simulink model "AariaJoystickR2017a"  (R2017a)
settings: Solver=VariableStepAuto  StartTime=0.0  StopTime=inf  FixedStep=0.1  RelTol=1e-3  EnableMultiTasking=on
model workspace (MATLAB code in the model file):
  | my_a =1;
undefined symbols (not defined in the file or in its folder): AARIAENV, AARIAMAN, AARIASEN, Camera, sensor, Source_TS, X, Y, Z
libraries: sm_lib x723, nesl_utility x640, dspmathops x314, simulink x168, vrlib x2, powerlib_meascontrol x1, aerolibanimutils x1, aerolibutil x1
(part 2 of 26)

== system AariaJoystickR2017a/Tool ==
  Cam_vis : sm_lib/Body Elements/Solid  InertiaType=CalculateFromGeometry  Mass=0  MassUnits=kg  CenterOfMass=[0 0 0]  CenterOfMassUnits=m  MomentsOfInertia=[1 1 1]  MomentsOfInertiaUnits=kg*m^2  ProductsOfInertia=[1 1 1]  ProductsOfInertiaUnits=kg*m^2  DensityBased=off  Density=1000  DensityUnits=kg/m^3  DoExposeReferenceFrame=on  SerializedFrames=<Frames/>  GraphicType=FromGeometry  MarkerShape=Sphere  MarkerSize=10  GraphicVisPropType=SimpleVisualProperties  GraphicDiffuseColor=[0.5 0.5 0.5]  GraphicSpecularColor=[0.5 0.5 0.5 1.0]  GraphicAmbientColor=[0.15 0.15 0.15 1.0]  GraphicEmissiveColor=[0.0 0.0 0.0 1.0]  GraphicShininess=75  GraphicOpacity=1.0  GeometryShape=Sphere  RectangleSize=[1 1]  RectangleSizeUnits=m  BrickDimensions=[0.01 0.01 0.2]  BrickDimensionUnits=m  CylinderRadius=1  CylinderRadiusUnits=m  CylinderLength=1  CylinderLengthUnits=m  SphereRadius=0.02  SphereRadiusUnits=m  EllipsoidRadii=[1 1 1]  EllipsoidRadiiUnits=m  ExtrusionCrossSection=[1 1; -1 1; -1 -1; 1 -1]  ExtrusionCrossSectionUnits=m  ExtrusionLength=1  ExtrusionLengthUnits=m  PolygonNumSides=3  PolygonOuterRadius=1  PolygonOuterRadiusUnits=m  ExtGeomFileType=STEP  ExtGeomFileUnits=m  RevolutionCrossSection=[1 1; 1 -1; 2 -1; 2 1]  RevolutionCrossSectionUnits=m  RevolutionExtent=Full  RevolutionAngle=180  RevolutionAngleUnits=deg
  Camera : sm_lib/Frames and Transforms/Reference Frame
  Coord_ToolTip : sm_lib/Body Elements/Graphic  GraphicType=Marker  MarkerShape=Frame  MarkerSize=AARIAMAN.vis.coord_size  GraphicVisPropType=SimpleVisualProperties  GraphicDiffuseColor=[1.0 1.0 0.0]  GraphicSpecularColor=[0.5 0.5 0.5 1.0]  GraphicAmbientColor=[0.15 0.15 0.15 1.0]  GraphicEmissiveColor=[0.0 0.0 0.0 1.0]  GraphicShininess=75  GraphicOpacity=1.0
      settings: SourceProductName=Simscape Multibody
  IMU Tool : Subsystem  mask{nL=Link_number}
      mask prompts: nL "Link Number (nL)"
      mask DialogControl DescTextVar Prompt: A Set of IMUs for one body
  Mux : Mux  Inputs=2
  Rigid Transform : sm_lib/Frames and Transforms/Rigid Transform  TranslationMethod=None  TranslationStandardOffset=0  TranslationLengthUnit=m  TranslationStandardAxis=+Z  TranslationCartesianOffset=[0 0 0]  TranslationROffset=0  TranslationROffsetUnits=m  TranslationZOffset=0  TranslationZOffsetUnits=m  TranslationThetaOffset=0  TranslationThetaOffsetUnits=deg  RotationMethod=AlignedAxes  RotationAngleUnits=deg  RotationStandardAxis=+Z  RotationAngle=0.0  RotationArbitraryAxis=[0 0 1]  FollAlignAxisA=+X  BaseAlignAxisA=+Z  FollAlignAxisB=+Z  BaseAlignAxisB=+Y  RotationSequenceAxes=FollowerAxes  RotationSequence=XYX  RotationSequenceAngles=[0 0 0]  RotationSequenceAnglesUnits=deg  RotationMatrix=[1 0 0; 0 1 0; 0 0 1]
  Rigid Transform1 : sm_lib/Frames and Transforms/Rigid Transform  TranslationMethod=StandardAxis  TranslationStandardOffset=AARIAMAN.DH(Link_number).a/2  TranslationLengthUnit=m  TranslationStandardAxis=+Z  TranslationCartesianOffset=0.1  TranslationROffset=0  TranslationROffsetUnits=m  TranslationZOffset=0  TranslationZOffsetUnits=m  TranslationThetaOffset=0  TranslationThetaOffsetUnits=deg  RotationMethod=None  RotationAngleUnits=deg  RotationStandardAxis=+Z  RotationAngle=0.0  RotationArbitraryAxis=[0 0 1]  FollAlignAxisA=+X  BaseAlignAxisA=+Y  FollAlignAxisB=+Y  BaseAlignAxisB=+Z  RotationSequenceAxes=FollowerAxes  RotationSequence=XYX  RotationSequenceAngles=[0 0 0]  RotationSequenceAnglesUnits=deg  RotationMatrix=[1 0 0; 0 1 0; 0 0 1]
  Rigid Transform2 : sm_lib/Frames and Transforms/Rigid Transform  TranslationMethod=StandardAxis  TranslationStandardOffset=AARIAMAN.DH(Link_number).a/2  TranslationLengthUnit=m  TranslationStandardAxis=+Z  TranslationCartesianOffset=0.1  TranslationROffset=0  TranslationROffsetUnits=m  TranslationZOffset=0  TranslationZOffsetUnits=m  TranslationThetaOffset=0  TranslationThetaOffsetUnits=deg  RotationMethod=None  RotationAngleUnits=deg  RotationStandardAxis=+Z  RotationAngle=0.0  RotationArbitraryAxis=[0 0 1]  FollAlignAxisA=+X  BaseAlignAxisA=+Y  FollAlignAxisB=+Y  BaseAlignAxisB=+Z  RotationSequenceAxes=FollowerAxes  RotationSequence=XYX  RotationSequenceAngles=[0 0 0]  RotationSequenceAnglesUnits=deg  RotationMatrix=[1 0 0; 0 1 0; 0 0 1]
  Rigid Transform3 : sm_lib/Frames and Transforms/Rigid Transform  TranslationMethod=StandardAxis  TranslationStandardOffset=AARIAMAN.DH(Link_number).d-0.01  TranslationLengthUnit=m  TranslationStandardAxis=-X  TranslationCartesianOffset=0.1  TranslationROffset=0  TranslationROffsetUnits=m  TranslationZOffset=0  TranslationZOffsetUnits=m  TranslationThetaOffset=0  TranslationThetaOffsetUnits=deg  RotationMethod=None  RotationAngleUnits=deg  RotationStandardAxis=+Z  RotationAngle=0.0  RotationArbitraryAxis=[0 0 1]  FollAlignAxisA=+X  BaseAlignAxisA=+Y  FollAlignAxisB=+Y  BaseAlignAxisB=+Z  RotationSequenceAxes=FollowerAxes  RotationSequence=XYX  RotationSequenceAngles=[0 0 0]  RotationSequenceAnglesUnits=deg  RotationMatrix=[1 0 0; 0 1 0; 0 0 1]
  Rigid Transform4 : sm_lib/Frames and Transforms/Rigid Transform  TranslationMethod=None  TranslationStandardOffset=0  TranslationLengthUnit=m  TranslationStandardAxis=+Z  TranslationCartesianOffset=[0 0 0]  TranslationROffset=0  TranslationROffsetUnits=m  TranslationZOffset=0  TranslationZOffsetUnits=m  TranslationThetaOffset=0  TranslationThetaOffsetUnits=deg  RotationMethod=AlignedAxes  RotationAngleUnits=deg  RotationStandardAxis=+Z  RotationAngle=0.0  RotationArbitraryAxis=[0 0 1]  FollAlignAxisA=+X  BaseAlignAxisA=+Z  FollAlignAxisB=+Z  BaseAlignAxisB=+Y  RotationSequenceAxes=FollowerAxes  RotationSequence=XYX  RotationSequenceAngles=[0 0 0]  RotationSequenceAnglesUnits=deg  RotationMatrix=[1 0 0; 0 1 0; 0 0 1]
  Rigid Transform5 : sm_lib/Frames and Transforms/Rigid Transform  TranslationMethod=None  TranslationStandardOffset=0.1  TranslationLengthUnit=m  TranslationStandardAxis=+Y  TranslationCartesianOffset=[0 0 0]  TranslationROffset=0  TranslationROffsetUnits=m  TranslationZOffset=0  TranslationZOffsetUnits=m  TranslationThetaOffset=0  TranslationThetaOffsetUnits=deg  RotationMethod=RotationMatrix  RotationAngleUnits=rad  RotationStandardAxis=+X  RotationAngle=Camera.Rotation  RotationArbitraryAxis=[0 0 1]  FollAlignAxisA=+X  BaseAlignAxisA=+Y  FollAlignAxisB=+Y  BaseAlignAxisB=+Z  RotationSequenceAxes=FollowerAxes  RotationSequence=XYX  RotationSequenceAngles=[0 0 0]  RotationSequenceAnglesUnits=deg  RotationMatrix=Camera.Rotation
  Rigid Transform7 : sm_lib/Frames and Transforms/Rigid Transform  TranslationMethod=Cartesian  TranslationStandardOffset=0.1  TranslationLengthUnit=m  TranslationStandardAxis=+Y  TranslationCartesianOffset=Camera.Offset  TranslationROffset=0  TranslationROffsetUnits=m  TranslationZOffset=0  TranslationZOffsetUnits=m  TranslationThetaOffset=0  TranslationThetaOffsetUnits=deg  RotationMethod=None  RotationAngleUnits=rad  RotationStandardAxis=+X  RotationAngle=Camera.Rotation  RotationArbitraryAxis=[0 0 1]  FollAlignAxisA=+X  BaseAlignAxisA=+Y  FollAlignAxisB=+Y  BaseAlignAxisB=+Z  RotationSequenceAxes=FollowerAxes  RotationSequence=XYX  RotationSequenceAngles=[0 0 0]  RotationSequenceAnglesUnits=deg  RotationMatrix=[1 0 0; 0 1 0; 0 0 1]
  Rigid Transform8 : sm_lib/Frames and Transforms/Rigid Transform  TranslationMethod=StandardAxis  TranslationStandardOffset=Camera.ObjectRadius  TranslationLengthUnit=m  TranslationStandardAxis=+Z  TranslationCartesianOffset=Camera.Offset  TranslationROffset=0  TranslationROffsetUnits=m  TranslationZOffset=0  TranslationZOffsetUnits=m  TranslationThetaOffset=0  TranslationThetaOffsetUnits=deg  RotationMethod=None  RotationAngleUnits=deg  RotationStandardAxis=+X  RotationAngle=-90  RotationArbitraryAxis=[0 0 1]  FollAlignAxisA=+X  BaseAlignAxisA=+Y  FollAlignAxisB=+Y  BaseAlignAxisB=+Z  RotationSequenceAxes=FollowerAxes  RotationSequence=XYX  RotationSequenceAngles=[0 0 0]  RotationSequenceAnglesUnits=deg  RotationMatrix=0
  Rigid Transform9 : sm_lib/Frames and Transforms/Rigid Transform  TranslationMethod=StandardAxis  TranslationStandardOffset=AARIAMAN.DH(Link_number).d-0.01  TranslationLengthUnit=m  TranslationStandardAxis=+X  TranslationCartesianOffset=0.1  TranslationROffset=0  TranslationROffsetUnits=m  TranslationZOffset=0  TranslationZOffsetUnits=m  TranslationThetaOffset=0  TranslationThetaOffsetUnits=deg  RotationMethod=None  RotationAngleUnits=deg  RotationStandardAxis=+Z  RotationAngle=0.0  RotationArbitraryAxis=[0 0 1]  FollAlignAxisA=+X  BaseAlignAxisA=+Y  FollAlignAxisB=+Y  BaseAlignAxisB=+Z  RotationSequenceAxes=FollowerAxes  RotationSequence=XYX  RotationSequenceAngles=[0 0 0]  RotationSequenceAnglesUnits=deg  RotationMatrix=[1 0 0; 0 1 0; 0 0 1]
  Terminator : Terminator
  Terminator1 : Terminator
  ToDH : sm_lib/Frames and Transforms/Rigid Transform  TranslationMethod=None  TranslationStandardOffset=0  TranslationLengthUnit=m  TranslationStandardAxis=+Z  TranslationCartesianOffset=[0 0 0]  TranslationROffset=0  TranslationROffsetUnits=m  TranslationZOffset=0  TranslationZOffsetUnits=m  TranslationThetaOffset=0  TranslationThetaOffsetUnits=deg  RotationMethod=RotationMatrix  RotationAngleUnits=deg  RotationStandardAxis=+Z  RotationAngle=0.0  RotationArbitraryAxis=[0 0 1]  FollAlignAxisA=+X  BaseAlignAxisA=+Y  FollAlignAxisB=+Y  BaseAlignAxisB=+Z  RotationSequenceAxes=FollowerAxes  RotationSequence=XYX  RotationSequenceAngles=[0 0 0]  RotationSequenceAnglesUnits=deg  RotationMatrix=AARIAMAN.L(Link_number).toDH
  Tool : sm_lib/Body Elements/Solid  InertiaType=CalculateFromGeometry  Mass=abs(AARIAMAN.L(Link_number).massLink)  MassUnits=kg  CenterOfMass=[0 0 0]  CenterOfMassUnits=m  MomentsOfInertia=[1 1 1]  MomentsOfInertiaUnits=kg*m^2  ProductsOfInertia=[0 0 0]  ProductsOfInertiaUnits=kg*m^2  DensityBased=off  Density=1000  DensityUnits=kg/(m^3)  DoExposeReferenceFrame=on  SerializedFrames=<Frames/>  GraphicType=FromGeometry  MarkerShape=Sphere  MarkerSize=10  GraphicVisPropType=SimpleVisualProperties  GraphicDiffuseColor=[0.6 0.0 0.0]  GraphicSpecularColor=[0.5 0.5 0.5 1.0]  GraphicAmbientColor=[0.15 0.15 0.15 1.0]  GraphicEmissiveColor=[0.0 0.0 0.0 1.0]  GraphicShininess=75  GraphicOpacity=AARIAMAN.L(Link_number).linkOpacity  GeometryShape=Cylinder  RectangleSize=[1 1]  RectangleSizeUnits=m  BrickDimensions=[1 1 1]  BrickDimensionUnits=m  CylinderRadius=abs(AARIAMAN.DH(Link_number).d)+0.001  CylinderRadiusUnits=m  CylinderLength=AARIAMAN.DH(Link_number).a+0.001  CylinderLengthUnits=m  SphereRadius=1  SphereRadiusUnits=m  EllipsoidRadii=[1 1 1]  EllipsoidRadiiUnits=m  ExtrusionCrossSection=[1 1; -1 1; -1 -1; 1 -1]  ExtrusionCrossSectionUnits=m  ExtrusionLength=1  ExtrusionLengthUnits=m  PolygonNumSides=3  PolygonOuterRadius=1  PolygonOuterRadiusUnits=m  ExtGeomFileType=STL  ExtGeomFileUnits=m  RevolutionCrossSection=[1 1; 1 -1; 2 -1; 2 1]  RevolutionCrossSectionUnits=m  RevolutionExtent=Full  RevolutionAngle=180  RevolutionAngleUnits=deg
  Tool1 : sm_lib/Body Elements/Solid  InertiaType=CalculateFromGeometry  Mass=AARIAMAN.vis.joint_mass/10  MassUnits=kg  CenterOfMass=[0 0 0]  CenterOfMassUnits=m  MomentsOfInertia=[1 1 1]  MomentsOfInertiaUnits=kg*m^2  ProductsOfInertia=[0 0 0]  ProductsOfInertiaUnits=kg*m^2  DensityBased=off  Density=1000  DensityUnits=kg/(m^3)  DoExposeReferenceFrame=on  SerializedFrames=<Frames/>  GraphicType=FromGeometry  MarkerShape=Sphere  MarkerSize=10  GraphicVisPropType=SimpleVisualProperties  GraphicDiffuseColor=[0.6 0.0 0.0]  GraphicSpecularColor=[0.5 0.5 0.5 1.0]  GraphicAmbientColor=[0.15 0.15 0.15 1.0]  GraphicEmissiveColor=[0.0 0.0 0.0 1.0]  GraphicShininess=75  GraphicOpacity=1.0  GeometryShape=Brick  RectangleSize=[1 1]  RectangleSizeUnits=m  BrickDimensions=[0.01 0.1 0.1]  BrickDimensionUnits=m  CylinderRadius=1  CylinderRadiusUnits=m  CylinderLength=1  CylinderLengthUnits=m  SphereRadius=1  SphereRadiusUnits=m  EllipsoidRadii=[1 1 1]  EllipsoidRadiiUnits=m  ExtrusionCrossSection=[1 1; -1 1; -1 -1; 1 -1]  ExtrusionCrossSectionUnits=m  ExtrusionLength=1  ExtrusionLengthUnits=m  PolygonNumSides=4  PolygonOuterRadius=1  PolygonOuterRadiusUnits=m  ExtGeomFileType=STL  ExtGeomFileUnits=m  RevolutionCrossSection=[1 1; 1 -1; 2 -1; 2 1]  RevolutionCrossSectionUnits=m  RevolutionExtent=Full  RevolutionAngle=180  RevolutionAngleUnits=deg
  Tool2 : sm_lib/Body Elements/Solid  InertiaType=CalculateFromGeometry  Mass=AARIAMAN.vis.joint_mass/10  MassUnits=kg  CenterOfMass=[0 0 0]  CenterOfMassUnits=m  MomentsOfInertia=[1 1 1]  MomentsOfInertiaUnits=kg*m^2  ProductsOfInertia=[0 0 0]  ProductsOfInertiaUnits=kg*m^2  DensityBased=off  Density=1000  DensityUnits=kg/(m^3)  DoExposeReferenceFrame=on  SerializedFrames=<Frames/>  GraphicType=FromGeometry  MarkerShape=Sphere  MarkerSize=10  GraphicVisPropType=SimpleVisualProperties  GraphicDiffuseColor=[0.6 0.0 0.0]  GraphicSpecularColor=[0.5 0.5 0.5 1.0]  GraphicAmbientColor=[0.15 0.15 0.15 1.0]  GraphicEmissiveColor=[0.0 0.0 0.0 1.0]  GraphicShininess=75  GraphicOpacity=1.0  GeometryShape=Brick  RectangleSize=[1 1]  RectangleSizeUnits=m  BrickDimensions=[0.01 0.1 0.1]  BrickDimensionUnits=m  CylinderRadius=1  CylinderRadiusUnits=m  CylinderLength=1  CylinderLengthUnits=m  SphereRadius=1  SphereRadiusUnits=m  EllipsoidRadii=[1 1 1]  EllipsoidRadiiUnits=m  ExtrusionCrossSection=[1 1; -1 1; -1 -1; 1 -1]  ExtrusionCrossSectionUnits=m  ExtrusionLength=1  ExtrusionLengthUnits=m  PolygonNumSides=4  PolygonOuterRadius=1  PolygonOuterRadiusUnits=m  ExtGeomFileType=STL  ExtGeomFileUnits=m  RevolutionCrossSection=[1 1; 1 -1; 2 -1; 2 1]  RevolutionCrossSectionUnits=m  RevolutionExtent=Full  RevolutionAngle=180  RevolutionAngleUnits=deg
  force_torque_sensor : Subsystem
  Base : PMIOPort  Port=1  Side=Left
  Reference : PMIOPort  Port=2  Side=Left
  Cam : PMIOPort  Port=3  Side=Right
  ToolTip : PMIOPort  Port=4  Side=Right
  Out1 : Outport
  Tool_torque : Outport  Port=2
  wires:
  IMU Tool/1(Out1) -> Mux/1
  IMU Tool/2(Out2) -> Mux/2
  Mux/1 -> Out1/1
  IMU Tool/3(Out3) -> Terminator/1
  IMU Tool/4(Out4) -> Terminator1/1
  force_torque_sensor/1(XYZ_force_torque) -> Tool_torque/1
  connections:
  Rigid Transform1/RConn1 -- Rigid Transform2/LConn1 -- Tool/RConn1
  IMU Tool/LConn2 -- Reference/RConn1
  ToDH/RConn1 -- Rigid Transform1/LConn1
  force_torque_sensor/LConn1 -- Base/RConn1
  force_torque_sensor/RConn1 -- ToDH/LConn1
  Rigid Transform9/LConn1 -- Rigid Transform3/LConn1 -- Rigid Transform7/LConn1 -- Rigid Transform8/LConn1 -- IMU Tool/LConn1 -- Rigid Transform2/RConn1
  Rigid Transform3/RConn1 -- Tool2/RConn1
  Tool1/RConn1 -- Rigid Transform9/RConn1
  Coord_ToolTip/RConn1 -- ToolTip/RConn1 -- Rigid Transform/RConn1
  Cam/RConn1 -- Rigid Transform5/RConn1 -- Cam_vis/RConn1 -- Camera/RConn1
  Rigid Transform/LConn1 -- Rigid Transform8/RConn1
  Rigid Transform4/RConn1 -- Rigid Transform5/LConn1
  Rigid Transform4/LConn1 -- Rigid Transform7/RConn1

== system AariaJoystickR2017a/Tool Sensors ==
  Camera sensor : Subsystem
  Object tracker : Subsystem
  Terminator{,1..5,8} (7 alike) : Terminator
  Tool sensor1 : Subsystem
  Tool sensor2 : Subsystem
  Camera : PMIOPort  Port=1  Side=Left
  ToolTip : PMIOPort  Port=2  Side=Left
  World : PMIOPort  Port=3  Side=Left
  Object : PMIOPort  Port=4  Side=Left
  cam2tip2sph : Outport
  SphericalRad : Outport  Port=2
  ObjPose : Outport  Port=3
  tipxyz1 : Outport  Port=4
  rot axis : Outport  Port=5
  Rmat : Outport  Port=6
  Omega : Outport  Port=7
  wires:
  Camera sensor/1(Out3) -> Object tracker/1(CamRotation)
  Tool sensor2/3(Out2) -> cam2tip2sph/1
  Camera sensor/2(Out1) -> Terminator/1
  Camera sensor/3(Out2) -> Terminator1/1
  Tool sensor2/1(Out3) -> Terminator2/1
  Tool sensor2/2(Out1) -> Terminator3/1
  Object tracker/1(Spherical Rad) -> SphericalRad/1
  Object tracker/2(Obj_pose) -> ObjPose/1
  Object tracker/3(Obj_pose_world) -> Terminator4/1
  Object tracker/4(xyz_true) -> Terminator5/1
  Tool sensor1/2(Out1) -> tipxyz1/1
  Tool sensor1/1(Out3) -> Rmat/1
  Tool sensor1/3(Out2) -> Terminator8/1
  Tool sensor1/4(rot axis) -> rot axis/1
  Tool sensor1/5(Omega) -> Omega/1
  connections:
  World/RConn1 -- Tool sensor1/LConn2 -- Camera sensor/LConn2
  Camera/RConn1 -- Tool sensor2/LConn2 -- Object tracker/LConn1 -- Camera sensor/LConn1
  Object/RConn1 -- Object tracker/RConn1
  Tool sensor2/LConn1 -- Tool sensor1/LConn1 -- ToolTip/RConn1

== system AariaJoystickR2017a/Base/BaseVSS ==
  BaseEmpty : Subsystem  VariantControl=VSS_MODE8 == 0
  BaseMotion : Subsystem  VariantControl=VSS_MODE8 == 1
  BaseTorque : Subsystem  VariantControl=VSS_MODE8 == 2
  Start : PMIOPort  Port=1  Side=Left
  End : PMIOPort  Port=2  Side=Right
  IMU : Outport

== system AariaJoystickR2017a/Joint1/JointVSS ==
  Control : Inport
  Empty : Subsystem  VariantControl=VSS_MODE1 == 0
  PrismaticMotion : Subsystem  VariantControl=VSS_MODE1 == 2
  PrismaticTorque : Subsystem  VariantControl=VSS_MODE1 == 4
  RevoluteMotion : Subsystem  VariantControl=VSS_MODE1 == 1
  RevoluteTorque : Subsystem  VariantControl=VSS_MODE1 == 3
  Start : PMIOPort  Port=1  Side=Left
  End : PMIOPort  Port=2  Side=Right
  Reference coord : PMIOPort  Port=3  Side=Left
  IMU : Outport
  Joint : Outport  Port=2

== system AariaJoystickR2017a/Joint2/JointVSS ==
  Control : Inport
  Empty : Subsystem  VariantControl=VSS_MODE2 == 0
  PrismaticMotion : Subsystem  VariantControl=VSS_MODE2 == 2
  PrismaticTorque : Subsystem  VariantControl=VSS_MODE2 == 4
  RevoluteMotion : Subsystem  VariantControl=VSS_MODE2 == 1
  RevoluteTorque : Subsystem  VariantControl=VSS_MODE2 == 3
  Start : PMIOPort  Port=1  Side=Left
  End : PMIOPort  Port=2  Side=Right
  Reference coord : PMIOPort  Port=3  Side=Left
  IMU : Outport
  Joint : Outport  Port=2

== system AariaJoystickR2017a/Joint3/JointVSS ==
  Control : Inport
  Empty : Subsystem  VariantControl=VSS_MODE3 == 0
  PrismaticMotion : Subsystem  VariantControl=VSS_MODE3 == 2
  PrismaticTorque : Subsystem  VariantControl=VSS_MODE3 == 4
  RevoluteMotion : Subsystem  VariantControl=VSS_MODE3 == 1
  RevoluteTorque : Subsystem  VariantControl=VSS_MODE3 == 3
  Start : PMIOPort  Port=1  Side=Left
  End : PMIOPort  Port=2  Side=Right
  Reference coord : PMIOPort  Port=3  Side=Left
  IMU : Outport
  Joint : Outport  Port=2

== system AariaJoystickR2017a/Joint4/JointVSS ==
  Control : Inport
  Empty : Subsystem  VariantControl=VSS_MODE4 == 0
  PrismaticMotion : Subsystem  VariantControl=VSS_MODE4 == 2
  PrismaticTorque : Subsystem  VariantControl=VSS_MODE4 == 4
  RevoluteMotion : Subsystem  VariantControl=VSS_MODE4 == 1
  RevoluteTorque : Subsystem  VariantControl=VSS_MODE4 == 3
  Start : PMIOPort  Port=1  Side=Left
  End : PMIOPort  Port=2  Side=Right
  Reference coord : PMIOPort  Port=3  Side=Left
  IMU : Outport
  Joint : Outport  Port=2

== system AariaJoystickR2017a/Joint5/JointVSS ==
  Control : Inport
  Empty : Subsystem  VariantControl=VSS_MODE5 == 0
  PrismaticMotion : Subsystem  VariantControl=VSS_MODE5 == 2
  PrismaticTorque : Subsystem  VariantControl=VSS_MODE5 == 4
  RevoluteMotion : Subsystem  VariantControl=VSS_MODE5 == 1
  RevoluteTorque : Subsystem  VariantControl=VSS_MODE5 == 3
  Start : PMIOPort  Port=1  Side=Left
  End : PMIOPort  Port=2  Side=Right
  Reference coord : PMIOPort  Port=3  Side=Left
  IMU : Outport
  Joint : Outport  Port=2

== system AariaJoystickR2017a/Joint6/JointVSS ==
  Control : Inport
  Empty : Subsystem  VariantControl=VSS_MODE6 == 0
  PrismaticMotion : Subsystem  VariantControl=VSS_MODE6 == 2
  PrismaticTorque : Subsystem  VariantControl=VSS_MODE6 == 4
  RevoluteMotion : Subsystem  VariantControl=VSS_MODE6 == 1
  RevoluteTorque : Subsystem  VariantControl=VSS_MODE6 == 3
  Start : PMIOPort  Port=1  Side=Left
  End : PMIOPort  Port=2  Side=Right
  Reference coord : PMIOPort  Port=3  Side=Left
  IMU : Outport
  Joint : Outport  Port=2

== system AariaJoystickR2017a/JoystickInputs/Variant Subsystem ==
  note: 1) Add Subsystem or Model blocks as valid variant choices.
      | 2) You cannot connect blocks at this level. At simulation, connectivity is automatically
      | determined, based on the active variant and port name matching.
  VSS_Live : Subsystem  VariantControl=VSS_Joystick == 1
  VSS_Replay : Subsystem  VariantControl=VSS_Joystick == 2
  Out1 : Outport
  Out2 : Outport  Port=2
  Out3 : Outport  Port=3
  Out4 : Outport  Port=4
  Out5 : Outport  Port=5
  Out6 : Outport  Port=6
  Out7 : Outport  Port=7

== system AariaJoystickR2017a/JoystickInputs/Variant Subsystem1 ==
  note: 1) Add Subsystem or Model blocks as valid variant choices.
      | 2) You cannot connect blocks at this level. At simulation, connectivity is automatically
      | determined, based on the active variant and port name matching.
  VSS_Live : Subsystem  VariantControl=VSS_Joystick == 1
  VSS_Replay : Subsystem  VariantControl=VSS_Joystick == 2
  Out1 : Outport
  Out2 : Outport  Port=2
  Out3 : Outport  Port=3
  Out4 : Outport  Port=4
  Out5 : Outport  Port=5
  Out6 : Outport  Port=6
  Out7 : Outport  Port=7

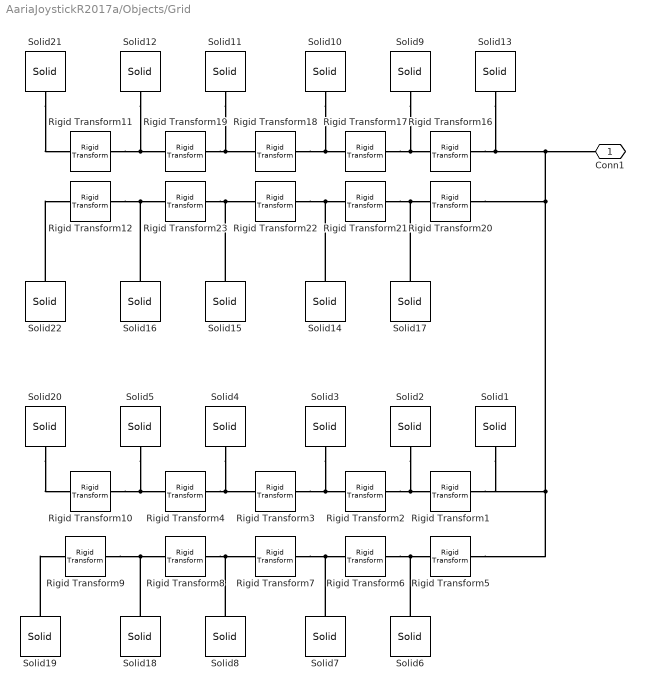
== system AariaJoystickR2017a/Objects/Grid ==
  Rigid Transform{1..4,10} (5 alike) : sm_lib/Frames and Transforms/Rigid Transform  TranslationMethod=StandardAxis  TranslationStandardOffset=2  TranslationLengthUnit=m  TranslationStandardAxis=+Y  TranslationCartesianOffset=[0 0 0]  TranslationROffset=0  TranslationROffsetUnits=m  TranslationZOffset=0  TranslationZOffsetUnits=m  TranslationThetaOffset=0  TranslationThetaOffsetUnits=deg  RotationMethod=None  RotationAngleUnits=deg  RotationStandardAxis=+Z  RotationAngle=0.0  RotationArbitraryAxis=[0 0 1]  FollAlignAxisA=+X  BaseAlignAxisA=+Y  FollAlignAxisB=+Y  BaseAlignAxisB=+Z  RotationSequenceAxes=FollowerAxes  RotationSequence=XYX  RotationSequenceAngles=[0 0 0]  RotationSequenceAnglesUnits=deg  RotationMatrix=[1 0 0; 0 1 0; 0 0 1]
  Rigid Transform{11,16..19} (5 alike) : sm_lib/Frames and Transforms/Rigid Transform  TranslationMethod=StandardAxis  TranslationStandardOffset=2  TranslationLengthUnit=m  TranslationStandardAxis=+X  TranslationCartesianOffset=[0 0 0]  TranslationROffset=0  TranslationROffsetUnits=m  TranslationZOffset=0  TranslationZOffsetUnits=m  TranslationThetaOffset=0  TranslationThetaOffsetUnits=deg  RotationMethod=None  RotationAngleUnits=deg  RotationStandardAxis=+Z  RotationAngle=0.0  RotationArbitraryAxis=[0 0 1]  FollAlignAxisA=+X  BaseAlignAxisA=+Y  FollAlignAxisB=+Y  BaseAlignAxisB=+Z  RotationSequenceAxes=FollowerAxes  RotationSequence=XYX  RotationSequenceAngles=[0 0 0]  RotationSequenceAnglesUnits=deg  RotationMatrix=[1 0 0; 0 1 0; 0 0 1]
  Rigid Transform{12,20..23} (5 alike) : sm_lib/Frames and Transforms/Rigid Transform  TranslationMethod=StandardAxis  TranslationStandardOffset=2  TranslationLengthUnit=m  TranslationStandardAxis=-X  TranslationCartesianOffset=[0 0 0]  TranslationROffset=0  TranslationROffsetUnits=m  TranslationZOffset=0  TranslationZOffsetUnits=m  TranslationThetaOffset=0  TranslationThetaOffsetUnits=deg  RotationMethod=None  RotationAngleUnits=deg  RotationStandardAxis=+Z  RotationAngle=0.0  RotationArbitraryAxis=[0 0 1]  FollAlignAxisA=+X  BaseAlignAxisA=+Y  FollAlignAxisB=+Y  BaseAlignAxisB=+Z  RotationSequenceAxes=FollowerAxes  RotationSequence=XYX  RotationSequenceAngles=[0 0 0]  RotationSequenceAnglesUnits=deg  RotationMatrix=[1 0 0; 0 1 0; 0 0 1]
  Rigid Transform{5..9} (5 alike) : sm_lib/Frames and Transforms/Rigid Transform  TranslationMethod=StandardAxis  TranslationStandardOffset=2  TranslationLengthUnit=m  TranslationStandardAxis=-Y  TranslationCartesianOffset=[0 0 0]  TranslationROffset=0  TranslationROffsetUnits=m  TranslationZOffset=0  TranslationZOffsetUnits=m  TranslationThetaOffset=0  TranslationThetaOffsetUnits=deg  RotationMethod=None  RotationAngleUnits=deg  RotationStandardAxis=+Z  RotationAngle=0.0  RotationArbitraryAxis=[0 0 1]  FollAlignAxisA=+X  BaseAlignAxisA=+Y  FollAlignAxisB=+Y  BaseAlignAxisB=+Z  RotationSequenceAxes=FollowerAxes  RotationSequence=XYX  RotationSequenceAngles=[0 0 0]  RotationSequenceAnglesUnits=deg  RotationMatrix=[1 0 0; 0 1 0; 0 0 1]
  Solid{1..8,18..20} (11 alike) : sm_lib/Body Elements/Solid  InertiaType=CalculateFromGeometry  Mass=1  MassUnits=kg  CenterOfMass=[0 0 0]  CenterOfMassUnits=m  MomentsOfInertia=[1 1 1]  MomentsOfInertiaUnits=kg*m^2  ProductsOfInertia=[1 1 1]  ProductsOfInertiaUnits=kg*m^2  DensityBased=on  Density=1000  DensityUnits=kg/m^3  DoExposeReferenceFrame=on  SerializedFrames=<Frames/>  GraphicType=FromGeometry  MarkerShape=Sphere  MarkerSize=10  GraphicVisPropType=SimpleVisualProperties  GraphicDiffuseColor=[0.4 0.4 0.4]  GraphicSpecularColor=[0.5 0.5 0.5 1.0]  GraphicAmbientColor=[0.15 0.15 0.15 1.0]  GraphicEmissiveColor=[0.0 0.0 0.0 1.0]  GraphicShininess=75  GraphicOpacity=1.0  GeometryShape=Brick  RectangleSize=[1 1]  RectangleSizeUnits=m  BrickDimensions=[20 1 0.12]  BrickDimensionUnits=m  CylinderRadius=1  CylinderRadiusUnits=m  CylinderLength=1  CylinderLengthUnits=m  SphereRadius=1  SphereRadiusUnits=m  EllipsoidRadii=[1 1 1]  EllipsoidRadiiUnits=m  ExtrusionCrossSection=[1 1; -1 1; -1 -1; 1 -1]  ExtrusionCrossSectionUnits=m  ExtrusionLength=1  ExtrusionLengthUnits=m  PolygonNumSides=3  PolygonOuterRadius=1  PolygonOuterRadiusUnits=m  ExtGeomFileType=STEP  ExtGeomFileUnits=m  RevolutionCrossSection=[1 1; 1 -1; 2 -1; 2 1]  RevolutionCrossSectionUnits=m  RevolutionExtent=Full  RevolutionAngle=180  RevolutionAngleUnits=deg
  Solid{9..17,21..22} (11 alike) : sm_lib/Body Elements/Solid  InertiaType=CalculateFromGeometry  Mass=1  MassUnits=kg  CenterOfMass=[0 0 0]  CenterOfMassUnits=m  MomentsOfInertia=[1 1 1]  MomentsOfInertiaUnits=kg*m^2  ProductsOfInertia=[1 1 1]  ProductsOfInertiaUnits=kg*m^2  DensityBased=on  Density=1000  DensityUnits=kg/m^3  DoExposeReferenceFrame=on  SerializedFrames=<Frames/>  GraphicType=FromGeometry  MarkerShape=Sphere  MarkerSize=10  GraphicVisPropType=SimpleVisualProperties  GraphicDiffuseColor=[0.2 0.2 0.2]  GraphicSpecularColor=[0.5 0.5 0.5 1.0]  GraphicAmbientColor=[0.15 0.15 0.15 1.0]  GraphicEmissiveColor=[0.0 0.0 0.0 1.0]  GraphicShininess=75  GraphicOpacity=1.0  GeometryShape=Brick  RectangleSize=[1 1]  RectangleSizeUnits=m  BrickDimensions=[1 20 0.11]  BrickDimensionUnits=m  CylinderRadius=1  CylinderRadiusUnits=m  CylinderLength=1  CylinderLengthUnits=m  SphereRadius=1  SphereRadiusUnits=m  EllipsoidRadii=[1 1 1]  EllipsoidRadiiUnits=m  ExtrusionCrossSection=[1 1; -1 1; -1 -1; 1 -1]  ExtrusionCrossSectionUnits=m  ExtrusionLength=1  ExtrusionLengthUnits=m  PolygonNumSides=3  PolygonOuterRadius=1  PolygonOuterRadiusUnits=m  ExtGeomFileType=STEP  ExtGeomFileUnits=m  RevolutionCrossSection=[1 1; 1 -1; 2 -1; 2 1]  RevolutionCrossSectionUnits=m  RevolutionExtent=Full  RevolutionAngle=180  RevolutionAngleUnits=deg
  Conn1 : PMIOPort  Port=1  Side=Right
  connections:
  Solid12/RConn1 -- Rigid Transform19/RConn1 -- Rigid Transform11/LConn1
  Rigid Transform19/LConn1 -- Solid11/RConn1 -- Rigid Transform18/RConn1
  Rigid Transform16/LConn1 -- Solid13/RConn1 -- Rigid Transform20/LConn1 -- Rigid Transform1/LConn1 -- Solid1/RConn1 -- Rigid Transform5/LConn1 -- Conn1/RConn1
  Rigid Transform21/LConn1 -- Solid17/RConn1 -- Rigid Transform20/RConn1
  Rigid Transform18/LConn1 -- Solid10/RConn1 -- Rigid Transform17/RConn1
  Rigid Transform23/LConn1 -- Rigid Transform22/RConn1 -- Solid15/RConn1
  Rigid Transform22/LConn1 -- Rigid Transform21/RConn1 -- Solid14/RConn1
  Rigid Transform17/LConn1 -- Solid9/RConn1 -- Rigid Transform16/RConn1
  Solid16/RConn1 -- Rigid Transform23/RConn1 -- Rigid Transform12/LConn1
  Rigid Transform2/LConn1 -- Solid2/RConn1 -- Rigid Transform1/RConn1
  Rigid Transform3/LConn1 -- Solid3/RConn1 -- Rigid Transform2/RConn1
  Rigid Transform4/LConn1 -- Rigid Transform3/RConn1 -- Solid4/RConn1
  Solid5/RConn1 -- Rigid Transform4/RConn1 -- Rigid Transform10/LConn1
  Rigid Transform6/LConn1 -- Solid6/RConn1 -- Rigid Transform5/RConn1
  Rigid Transform7/LConn1 -- Solid7/RConn1 -- Rigid Transform6/RConn1
  Rigid Transform8/LConn1 -- Rigid Transform7/RConn1 -- Solid8/RConn1
  Solid18/RConn1 -- Rigid Transform8/RConn1 -- Rigid Transform9/LConn1
  Solid19/RConn1 -- Rigid Transform9/RConn1
  Solid20/RConn1 -- Rigid Transform10/RConn1
  Solid21/RConn1 -- Rigid Transform11/RConn1
  Solid22/RConn1 -- Rigid Transform12/RConn1

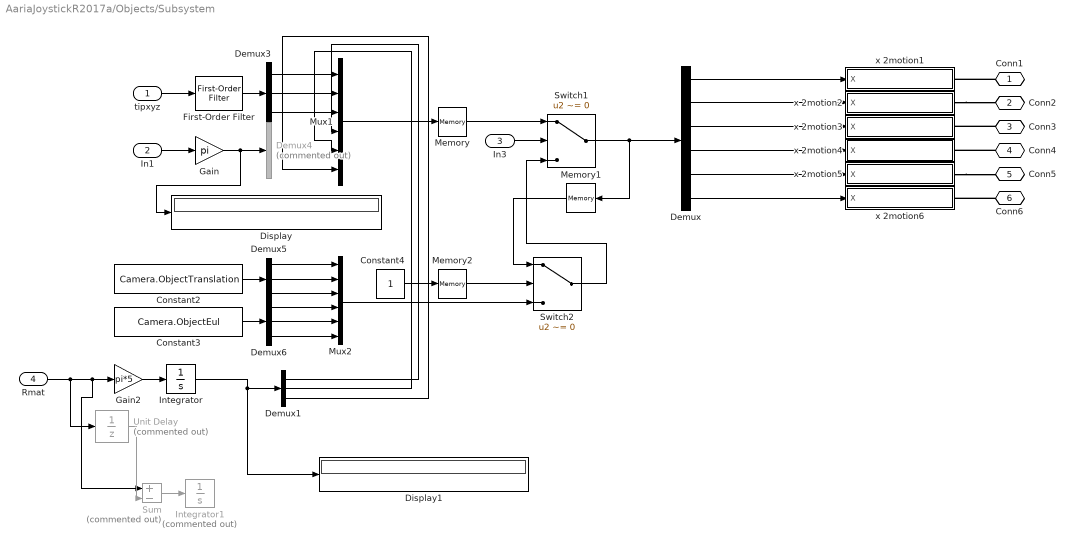
== system AariaJoystickR2017a/Objects/Subsystem ==
  tipxyz : Inport
  In1 : Inport  Port=2
  In3 : Inport  Port=3
  Rmat : Inport  Port=4
  Constant2 : Constant  Value=Camera.ObjectTranslation
  Constant3 : Constant  Value=Camera.ObjectEul
  Constant4 : Constant
  Demux : Demux  Outputs=6
  Demux{1,3,5..6} (4 alike) : Demux  Outputs=3
  Demux4 : Demux  Commented=on  Outputs=3
  Display : Display
  Display1 : Display
  First-Order Filter : powerlib_meascontrol/Filters/First-Order Filter  FilterType=Lowpass  Tc=10e-3  Ts=0  Initialize=on  Vac_Init=[0, 0, 60]  Vdc_Init=0  PlotResponse=off  FreqRange="[0,  200,  1]"
      settings: SourceProductName=Simscape Power Systems
  Gain : Gain  Gain=pi
  Gain2 : Gain  Gain=pi*5
  Integrator : Integrator
  Integrator1 : Integrator  Commented=on
  Memory : Memory
  Memory1 : Memory
  Memory2 : Memory
  Mux1 : Mux  Inputs=6
  Mux2 : Mux  Inputs=6
  Sum : Sum  Commented=on  Inputs=+-
  Switch1 : Switch  Criteria=u2 ~= 0
  Switch2 : Switch  Criteria=u2 ~= 0
  Unit Delay : UnitDelay  Commented=on  SampleTime=-1
  x 2motion1 : Subsystem
  x 2motion2 : Subsystem
  x 2motion3 : Subsystem
  x 2motion4 : Subsystem
  x 2motion5 : Subsystem
  x 2motion6 : Subsystem
  Conn1 : PMIOPort  Port=1  Side=Right
  Conn2 : PMIOPort  Port=2  Side=Right
  Conn3 : PMIOPort  Port=3  Side=Right
  Conn4 : PMIOPort  Port=4  Side=Right
  Conn5 : PMIOPort  Port=5  Side=Right
  Conn6 : PMIOPort  Port=6  Side=Right
  wires:
  Switch1/1 -> Memory1/1, Demux/1
  In3/1 -> Switch1/2
  tipxyz/1 -> First-Order Filter/1
  Demux/1 -> x 2motion1/1(X)
  Demux/2 -> x 2motion2/1(X)
  Demux/3 -> x 2motion3/1(X)
  Mux1/1 -> Memory/1
  First-Order Filter/1 -> Demux3/1
  Demux/4 -> x 2motion4/1(X)
  Demux/5 -> x 2motion5/1(X)
  Demux/6 -> x 2motion6/1(X)
  In1/1 -> Gain/1
  Memory1/1 -> Switch2/1
  Constant2/1 -> Demux5/1
  Constant3/1 -> Demux6/1
  Demux5/1 -> Mux2/1
  Demux5/2 -> Mux2/2
  Demux5/3 -> Mux2/3
  Demux6/3 -> Mux2/6
  Demux6/2 -> Mux2/5
  Demux6/1 -> Mux2/4
  Mux2/1 -> Switch2/3
  Switch2/1 -> Switch1/3
  Memory2/1 -> Switch2/2
  Constant4/1 -> Memory2/1
  Demux3/1 -> Mux1/1
  Demux3/2 -> Mux1/2
  Demux3/3 -> Mux1/3
  Memory/1 -> Switch1/1
  Gain/1 -> Display/1, Demux4/1
  Demux1/1 -> Mux1/4
  Demux1/2 -> Mux1/5
  Demux1/3 -> Mux1/6
  Rmat/1 -> Unit Delay/1, Sum/1, Gain2/1
  Integrator/1 -> Demux1/1, Display1/1
  Gain2/1 -> Integrator/1
  Unit Delay/1 -> Sum/2
  Sum/1 -> Integrator1/1
  connections:
  x 2motion2/RConn1 -- Conn2/RConn1
  Conn6/RConn1 -- x 2motion6/RConn1
  x 2motion5/RConn1 -- Conn5/RConn1
  Conn1/RConn1 -- x 2motion1/RConn1
  Conn3/RConn1 -- x 2motion3/RConn1
  Conn4/RConn1 -- x 2motion4/RConn1

== system AariaJoystickR2017a/Objects/Walls ==
  Grid : Subsystem
  Grid1 : Subsystem
  Grid2 : Subsystem
  Grid3 : Subsystem
  Rigid Transform{1,3,6,9} (4 alike) : sm_lib/Frames and Transforms/Rigid Transform  TranslationMethod=None  TranslationStandardOffset=10  TranslationLengthUnit=m  TranslationStandardAxis=+Y  TranslationCartesianOffset=[0 0 0]  TranslationROffset=0  TranslationROffsetUnits=m  TranslationZOffset=0  TranslationZOffsetUnits=m  TranslationThetaOffset=0  TranslationThetaOffsetUnits=deg  RotationMethod=StandardAxis  RotationAngleUnits=deg  RotationStandardAxis=+X  RotationAngle=90  RotationArbitraryAxis=[0 0 1]  FollAlignAxisA=+X  BaseAlignAxisA=+Y  FollAlignAxisB=+Y  BaseAlignAxisB=+Z  RotationSequenceAxes=FollowerAxes  RotationSequence=XYX  RotationSequenceAngles=[0 0 0]  RotationSequenceAnglesUnits=deg  RotationMatrix=[1 0 0; 0 1 0; 0 0 1]
  Rigid Transform10 : sm_lib/Frames and Transforms/Rigid Transform  TranslationMethod=StandardAxis  TranslationStandardOffset=10  TranslationLengthUnit=m  TranslationStandardAxis=-X  TranslationCartesianOffset=[0 0 0]  TranslationROffset=0  TranslationROffsetUnits=m  TranslationZOffset=0  TranslationZOffsetUnits=m  TranslationThetaOffset=0  TranslationThetaOffsetUnits=deg  RotationMethod=None  RotationAngleUnits=deg  RotationStandardAxis=+Z  RotationAngle=0.0  RotationArbitraryAxis=[0 0 1]  FollAlignAxisA=+X  BaseAlignAxisA=+Y  FollAlignAxisB=+Y  BaseAlignAxisB=+Z  RotationSequenceAxes=FollowerAxes  RotationSequence=XYX  RotationSequenceAngles=[0 0 0]  RotationSequenceAnglesUnits=deg  RotationMatrix=[1 0 0; 0 1 0; 0 0 1]
  Rigid Transform{2,5,8,11} (4 alike) : sm_lib/Frames and Transforms/Rigid Transform  TranslationMethod=StandardAxis  TranslationStandardOffset=4.5  TranslationLengthUnit=m  TranslationStandardAxis=+Y  TranslationCartesianOffset=[0 0 0]  TranslationROffset=0  TranslationROffsetUnits=m  TranslationZOffset=0  TranslationZOffsetUnits=m  TranslationThetaOffset=0  TranslationThetaOffsetUnits=deg  RotationMethod=None  RotationAngleUnits=deg  RotationStandardAxis=+Z  RotationAngle=0.0  RotationArbitraryAxis=[0 0 1]  FollAlignAxisA=+X  BaseAlignAxisA=+Y  FollAlignAxisB=+Y  BaseAlignAxisB=+Z  RotationSequenceAxes=FollowerAxes  RotationSequence=XYX  RotationSequenceAngles=[0 0 0]  RotationSequenceAnglesUnits=deg  RotationMatrix=[1 0 0; 0 1 0; 0 0 1]
  Rigid Transform12 : sm_lib/Frames and Transforms/Rigid Transform  TranslationMethod=None  TranslationStandardOffset=4.5  TranslationLengthUnit=m  TranslationStandardAxis=+Y  TranslationCartesianOffset=[0 0 0]  TranslationROffset=0  TranslationROffsetUnits=m  TranslationZOffset=0  TranslationZOffsetUnits=m  TranslationThetaOffset=0  TranslationThetaOffsetUnits=deg  RotationMethod=StandardAxis  RotationAngleUnits=deg  RotationStandardAxis=+Y  RotationAngle=90  RotationArbitraryAxis=[0 0 1]  FollAlignAxisA=+X  BaseAlignAxisA=+Y  FollAlignAxisB=+Y  BaseAlignAxisB=+Z  RotationSequenceAxes=FollowerAxes  RotationSequence=XYX  RotationSequenceAngles=[0 0 0]  RotationSequenceAnglesUnits=deg  RotationMatrix=[1 0 0; 0 1 0; 0 0 1]
  Rigid Transform13 : sm_lib/Frames and Transforms/Rigid Transform  TranslationMethod=None  TranslationStandardOffset=4.5  TranslationLengthUnit=m  TranslationStandardAxis=+Y  TranslationCartesianOffset=[0 0 0]  TranslationROffset=0  TranslationROffsetUnits=m  TranslationZOffset=0  TranslationZOffsetUnits=m  TranslationThetaOffset=0  TranslationThetaOffsetUnits=deg  RotationMethod=StandardAxis  RotationAngleUnits=deg  RotationStandardAxis=+Y  RotationAngle=90  RotationArbitraryAxis=[0 0 1]  FollAlignAxisA=+X  BaseAlignAxisA=+Y  FollAlignAxisB=+Y  BaseAlignAxisB=+Z  RotationSequenceAxes=FollowerAxes  RotationSequence=XYX  RotationSequenceAngles=[0 0 0]  RotationSequenceAnglesUnits=deg  RotationMatrix=[1 0 0; 0 1 0; 0 0 1]
  Rigid Transform16 : sm_lib/Frames and Transforms/Rigid Transform  TranslationMethod=StandardAxis  TranslationStandardOffset=10  TranslationLengthUnit=m  TranslationStandardAxis=+Y  TranslationCartesianOffset=[0 0 0]  TranslationROffset=0  TranslationROffsetUnits=m  TranslationZOffset=0  TranslationZOffsetUnits=m  TranslationThetaOffset=0  TranslationThetaOffsetUnits=deg  RotationMethod=None  RotationAngleUnits=deg  RotationStandardAxis=+Z  RotationAngle=0.0  RotationArbitraryAxis=[0 0 1]  FollAlignAxisA=+X  BaseAlignAxisA=+Y  FollAlignAxisB=+Y  BaseAlignAxisB=+Z  RotationSequenceAxes=FollowerAxes  RotationSequence=XYX  RotationSequenceAngles=[0 0 0]  RotationSequenceAnglesUnits=deg  RotationMatrix=[1 0 0; 0 1 0; 0 0 1]
  Rigid Transform4 : sm_lib/Frames and Transforms/Rigid Transform  TranslationMethod=StandardAxis  TranslationStandardOffset=10  TranslationLengthUnit=m  TranslationStandardAxis=-Y  TranslationCartesianOffset=[0 0 0]  TranslationROffset=0  TranslationROffsetUnits=m  TranslationZOffset=0  TranslationZOffsetUnits=m  TranslationThetaOffset=0  TranslationThetaOffsetUnits=deg  RotationMethod=None  RotationAngleUnits=deg  RotationStandardAxis=+Z  RotationAngle=0.0  RotationArbitraryAxis=[0 0 1]  FollAlignAxisA=+X  BaseAlignAxisA=+Y  FollAlignAxisB=+Y  BaseAlignAxisB=+Z  RotationSequenceAxes=FollowerAxes  RotationSequence=XYX  RotationSequenceAngles=[0 0 0]  RotationSequenceAnglesUnits=deg  RotationMatrix=[1 0 0; 0 1 0; 0 0 1]
  Rigid Transform7 : sm_lib/Frames and Transforms/Rigid Transform  TranslationMethod=StandardAxis  TranslationStandardOffset=10  TranslationLengthUnit=m  TranslationStandardAxis=+X  TranslationCartesianOffset=[0 0 0]  TranslationROffset=0  TranslationROffsetUnits=m  TranslationZOffset=0  TranslationZOffsetUnits=m  TranslationThetaOffset=0  TranslationThetaOffsetUnits=deg  RotationMethod=None  RotationAngleUnits=deg  RotationStandardAxis=+Z  RotationAngle=0.0  RotationArbitraryAxis=[0 0 1]  FollAlignAxisA=+X  BaseAlignAxisA=+Y  FollAlignAxisB=+Y  BaseAlignAxisB=+Z  RotationSequenceAxes=FollowerAxes  RotationSequence=XYX  RotationSequenceAngles=[0 0 0]  RotationSequenceAnglesUnits=deg  RotationMatrix=[1 0 0; 0 1 0; 0 0 1]
  Conn2 : PMIOPort  Port=1  Side=Left
  connections:
  Rigid Transform16/RConn1 -- Rigid Transform1/LConn1
  Rigid Transform16/LConn1 -- Rigid Transform10/LConn1 -- Rigid Transform7/LConn1 -- Rigid Transform4/LConn1 -- Conn2/RConn1
  Rigid Transform2/RConn1 -- Grid/RConn1
  Rigid Transform1/RConn1 -- Rigid Transform2/LConn1
  Rigid Transform3/RConn1 -- Rigid Transform5/LConn1
  Rigid Transform5/RConn1 -- Grid1/RConn1
  Rigid Transform4/RConn1 -- Rigid Transform3/LConn1
  Rigid Transform7/RConn1 -- Rigid Transform6/LConn1
  Rigid Transform8/RConn1 -- Grid2/RConn1
  Rigid Transform6/RConn1 -- Rigid Transform12/LConn1
  Rigid Transform13/RConn1 -- Rigid Transform11/LConn1
  Rigid Transform11/RConn1 -- Grid3/RConn1
  Rigid Transform10/RConn1 -- Rigid Transform9/LConn1
  Rigid Transform12/RConn1 -- Rigid Transform8/LConn1
  Rigid Transform9/RConn1 -- Rigid Transform13/LConn1

== system AariaJoystickR2017a/Subsystem/FoV ==
  spherical coord : Inport
  Covered : Inport  Port=2
  Abs : Abs
  Abs1 : Abs
  Constant : Constant  Value=Camera.horizontal_fov/2
  Constant1 : Constant  Value=Camera.vertical_fov/2
  Constant2 : Constant  Value=Camera.range
  Demux : Demux  Outputs=3
  Logical Operator1 : Logic  Operator=NOT  AllPortsSameDT=off  OutDataTypeStr=boolean
  Logical Operator2 : Logic  Inputs=4  AllPortsSameDT=off  OutDataTypeStr=boolean
  Relational Operator : RelationalOperator  OutDataTypeStr=boolean  RndMeth=Simplest
  Relational Operator1 : RelationalOperator  Operator=<=  OutDataTypeStr=boolean  RndMeth=Simplest
  Relational Operator2 : RelationalOperator  Operator=<=  OutDataTypeStr=boolean  RndMeth=Simplest
  Scope : Scope  NumInputPorts=3
  Scope1 : Scope  NumInputPorts=3
  Obj_visible : Outport
  wires:
  spherical coord/1 -> Demux/1
  Constant/1 -> Scope1/2, Relational Operator/1
  Demux/1 -> Abs/1
  Constant1/1 -> Relational Operator1/2
  Demux/3 -> Abs1/1
  Relational Operator1/1 -> Scope/3, Logical Operator2/3
  Relational Operator/1 -> Scope/1, Logical Operator2/1
  Abs/1 -> Scope1/1, Relational Operator/2
  Abs1/1 -> Scope1/3, Relational Operator1/1
  Demux/2 -> Relational Operator2/1
  Covered/1 -> Logical Operator1/1
  Logical Operator1/1 -> Logical Operator2/4
  Logical Operator2/1 -> Obj_visible/1
  Constant2/1 -> Relational Operator2/2
  Relational Operator2/1 -> Scope/2, Logical Operator2/2

== system AariaJoystickR2017a/Subsystem/Score ==
  In1 : Inport
  In2 : Inport  Port=2
  Data Type Conversion : DataTypeConversion  OutDataTypeStr=double
  Demux : Demux
  Gain : Gain
  Gain1 : Gain  Gain=100
  Gain2 : Gain  Gain=20
  Gain3 : Gain  Gain=30
  Gain4 : Gain  Gain=20
  Product : Product
  Saturation : Saturate  UpperLimit=100  LowerLimit=0
  Sum : Sum  Inputs=+++
  Sum1 : Sum
  Out1 : Outport
  Out2 : Outport  Port=2
  wires:
  In1/1 -> Data Type Conversion/1
  Demux/1 -> Gain/1  "vis"
  Demux/2 -> Gain1/1  "grab"
  Demux/3 -> Gain2/1  "pose"
  Demux/4 -> Gain3/1  "orient"
  Gain/1 -> Product/1
  Gain2/1 -> Sum/1
  Gain3/1 -> Sum/2
  Product/1 -> Sum1/2
  Data Type Conversion/1 -> Demux/1
  Sum/1 -> Product/2
  In2/1 -> Gain4/1
  Gain4/1 -> Sum/3
  Saturation/1 -> Out1/1
  Sum1/1 -> Out2/1, Saturation/1
  Gain1/1 -> Sum1/1

== system AariaJoystickR2017a/Subsystem/grab_check_cam above angled down ==
  note: compares spherical coordinates from tool to camera and camera to object (doesn't work always)
  note: compares spherical coordinates from camera to and camera to object
  CamObjSph : Inport
  ObjPose : Inport  Port=2
  TipCamSph : Inport  Port=3
  Logical Operator : Logic  AllPortsSameDT=off  OutDataTypeStr=boolean
  Subsystem : Subsystem
  Sum : Sum
  orientation match : Subsystem  Commented=on
  orientation match1 : Subsystem
  pose match : Subsystem
  grab ok : Outport
  pose ok : Outport  Port=2
  orientation ok : Outport  Port=3
  Bonus : Outport  Port=4  OutDataTypeStr=double
  wires:
  TipCamSph/1 -> orientation match1/1(TipCam)
  Subsystem/1(TipObjPose) -> pose match/1(Obj_pose)
  ObjPose/1 -> Subsystem/1(CamObj)
  CamObjSph/1 -> orientation match1/2(CamObj)
  pose match/1(grab_pose_ok) -> pose ok/1, Logical Operator/1
  Logical Operator/1 -> grab ok/1
  orientation match1/2(Orient_penalty) -> Sum/2
  pose match/2(PoseBonus) -> Sum/1
  Sum/1 -> Bonus/1
  orientation match1/1(Out1) -> orientation ok/1, Logical Operator/2

== system AariaJoystickR2017a/Subsystem2/Subsystem1 ==
  Trigger : TriggerPort  VariantControl=Variant  PortDimensions=1
  Constant : Constant
  Constant1 : Constant  Value=0
  Memory : Memory  InheritSampleTime=on
  Switch : Switch  Criteria=u2 > Threshold
  Out1 : Outport
  wires:
  Constant/1 -> Switch/3
  Switch/1 -> Out1/1, Memory/1
  Memory/1 -> Switch/2
  Constant1/1 -> Switch/1

== system AariaJoystickR2017a/Tool/IMU Tool ==
  Sensor Module1 : Subsystem  mask{nL=nL, nS=1}
      mask prompts: nL "Link Number"; nS "Sensor ID of that link"
      mask DialogControl DescGroupVar Prompt: Virtual IMU
      mask DialogControl DescTextVar Prompt: Measures Connected Body's acceleration and angular velocity in the given point
      mask DialogControl Control2 Prompt: The following numbers defines the corresponding numbers for this sensor to read from the parameters file
  Body Coord : PMIOPort  Port=1  Side=Left
  Reference Coord : PMIOPort  Port=2  Side=Left
  Out1 : Outport
  Out2 : Outport  Port=2
  Out3 : Outport  Port=3
  Out4 : Outport  Port=4
  wires:
  Sensor Module1/3(Out2) -> Out3/1
  Sensor Module1/2(Out4) -> Out2/1
  Sensor Module1/4(Out3) -> Out4/1
  Sensor Module1/1(Out5) -> Out1/1
  connections:
  Sensor Module1/LConn2 -- Reference Coord/RConn1
  Sensor Module1/LConn1 -- Body Coord/RConn1
